simulink model "exercise02_simulation_model_template_R2025b_Solution"  (R2025b)
settings: Solver=FixedStepAuto  StartTime=0.0  StopTime=10.0  FixedStep=1e-5  RelTol=1e-3
PreLoadFcn:
  | exercise02_simulation_parameters
undefined symbols (not defined in the file or in its folder): g, nrotor_initial_conditions, nrotor_vehicle, reference, sigbuilder_block
settings Model: Creator=resjoehr  LastModifiedBy=diego
settings DataIOCC: SaveFormat=Array  StreamToWks=off  ReturnWorkspaceOutputs=off

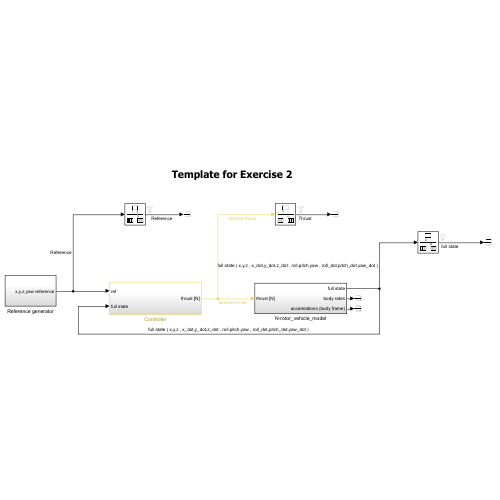
[thumbnail: Simulink's stored preview of the top-level diagram]
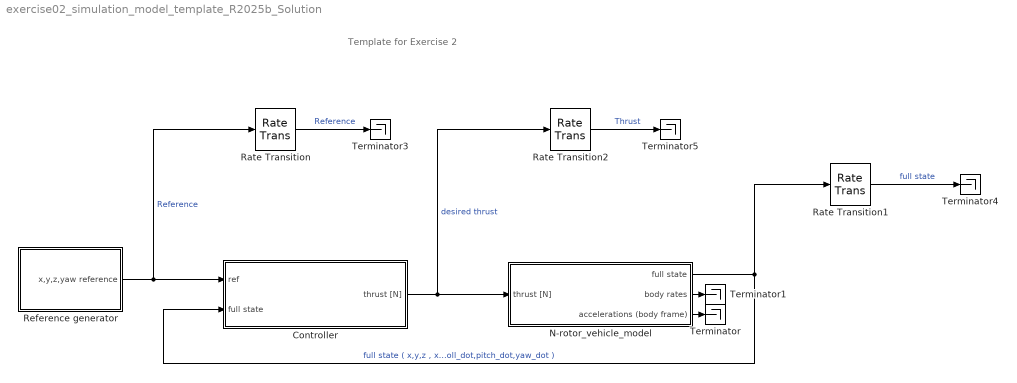
== system exercise02_simulation_model_template_R2025b_Solution ==
  note: Template for Exercise 2
  Controller : Subsystem
  N-rotor_vehicle_model : Subsystem
  Rate Transition : RateTransition  OutPortSampleTime=0.001
  Rate Transition1 : RateTransition  OutPortSampleTime=0.001
  Rate Transition2 : RateTransition  OutPortSampleTime=0.001
  Reference generator : Subsystem
  Terminator{,1,3..5} (5 alike) : Terminator
  wires:
  Rate Transition/1 -> Terminator3/1  "Reference"
  N-rotor_vehicle_model/2(body rates) -> Terminator1/1
  Reference generator/1(x,y,z,yaw reference) -> Rate Transition/1, Controller/1(ref)  "Reference"
  N-rotor_vehicle_model/1(full state) -> Rate Transition1/1, Controller/2(full state)  "full state ( x,y,z , x_dot,y_dot,z_dot , roll,pitch,yaw , roll_dot,pitch_dot,yaw_dot )"
  Rate Transition1/1 -> Terminator4/1  "full state"
  Rate Transition2/1 -> Terminator5/1  "Thrust"
  Controller/1(thrust [N]) -> N-rotor_vehicle_model/1(thrust [N]), Rate Transition2/1  "desired thrust"
  N-rotor_vehicle_model/3(accelerations (body frame)) -> Terminator/1

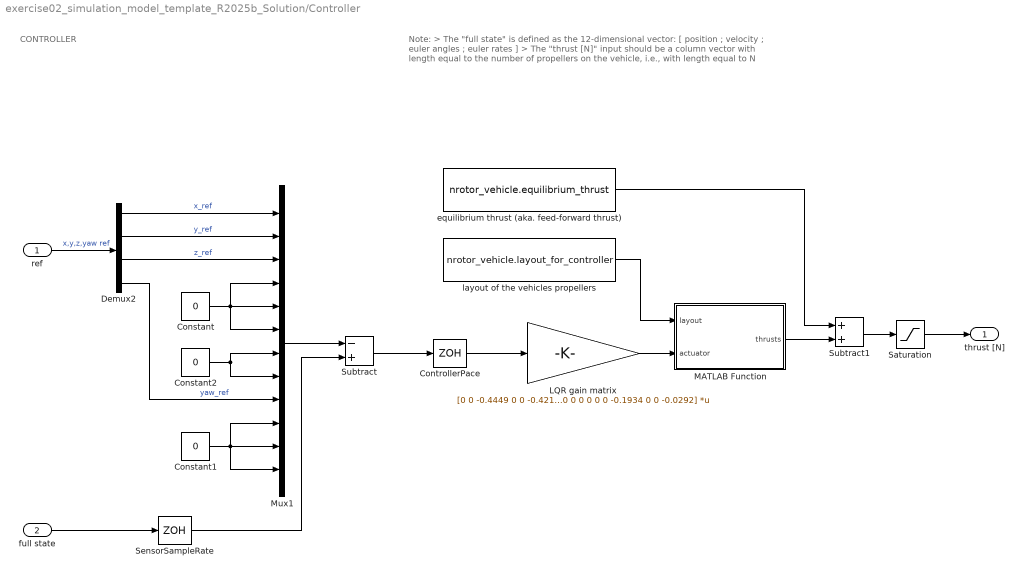
== system exercise02_simulation_model_template_R2025b_Solution/Controller ==
  note: CONTROLLER
  note: Note:
      | > The "full state" is defined as the 12-dimensional vector:
      | [ position ; velocity ; euler angles ; euler rates ]
      | > The "thrust [N]" input should be a column vector with
      | length equal to the number of propellers on the vehicle,
      | i.e., with length equal to N
  ref : Inport
  full state : Inport  Port=2
  Constant : Constant  Value=0
  Constant1 : Constant  Value=0
  Constant2 : Constant  Value=0
  ControllerPace : ZeroOrderHold  SampleTime=0.1
  Demux2 : Demux
  LQR gain matrix : Gain  Gain=[0 0 -0.4449 0 0 -0.4218 0 0 0 0 0 0;0 0.1322 0 0 0.1006 0 -0.3757 0 0 -0.0287 0 0;-0.1322 0 0 -0.1006 0 0 0 -0.3757 0 0 -0.0287 0;0 0 0 0 0 0 0 0 -0.1934 0 0 -0.0292]  Multiplication=Matrix(K*u)
  MATLAB Function : MATLAB Function  TreatAsAtomicUnit=on
  Mux1 : Mux  Inputs=12
  Saturation : Saturate  UpperLimit=nrotor_vehicle.thrust_max  LowerLimit=nrotor_vehicle.thrust_min  ZeroCross=off
  SensorSampleRate : ZeroOrderHold  SampleTime=0.005
  Subtract : Sum  Inputs=-+
  Subtract1 : Sum
  equilibrium thrust (aka. feed-forward thrust) : Constant  Value=nrotor_vehicle.equilibrium_thrust
  layout of the vehicles propellers : Constant  Value=nrotor_vehicle.layout_for_controller
  thrust [N] : Outport  VectorParamsAs1DForOutWhenUnconnected=off
  wires:
  Saturation/1 -> thrust [N]/1
  ref/1 -> Demux2/1  "x,y,z,yaw ref"
  Mux1/1 -> Subtract/1
  Demux2/1 -> Mux1/1  "x_ref"
  Demux2/2 -> Mux1/2  "y_ref"
  Demux2/3 -> Mux1/3  "z_ref"
  Constant/1 -> Mux1/6, Mux1/5, Mux1/4
  full state/1 -> SensorSampleRate/1
  Subtract/1 -> ControllerPace/1
  LQR gain matrix/1 -> MATLAB Function/2(actuator)
  Subtract1/1 -> Saturation/1
  equilibrium thrust (aka. feed-forward thrust)/1 -> Subtract1/1
  Constant1/1 -> Mux1/11, Mux1/12, Mux1/10
  Constant2/1 -> Mux1/8, Mux1/7
  Demux2/4 -> Mux1/9  "yaw_ref"
  MATLAB Function/1(thrusts) -> Subtract1/2
  layout of the vehicles propellers/1 -> MATLAB Function/1(layout)
  ControllerPace/1 -> LQR gain matrix/1
  SensorSampleRate/1 -> Subtract/2

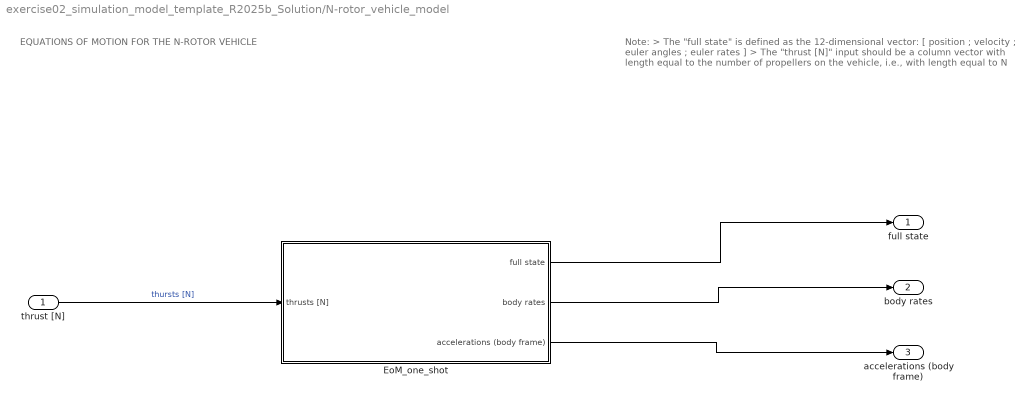
== system exercise02_simulation_model_template_R2025b_Solution/N-rotor_vehicle_model ==
  note: Note:
      | > The "full state" is defined as the 12-dimensional vector:
      | [ position ; velocity ; euler angles ; euler rates ]
      | > The "thrust [N]" input should be a column vector with
      | length equal to the number of propellers on the vehicle,
      | i.e., with length equal to N
  note: EQUATIONS OF MOTION FOR THE N-ROTOR VEHICLE
  thrust [N] : Inport
  EoM_one_shot : Subsystem
  full state : Outport  VectorParamsAs1DForOutWhenUnconnected=off
  body rates : Outport  Port=2  VectorParamsAs1DForOutWhenUnconnected=off
  accelerations (body frame) : Outport  Port=3  VectorParamsAs1DForOutWhenUnconnected=off
  wires:
  thrust [N]/1 -> EoM_one_shot/1(thrusts [N])  "thursts [N]"
  EoM_one_shot/1(full state) -> full state/1
  EoM_one_shot/2(body rates) -> body rates/1
  EoM_one_shot/3(accelerations (body frame)) -> accelerations (body frame)/1

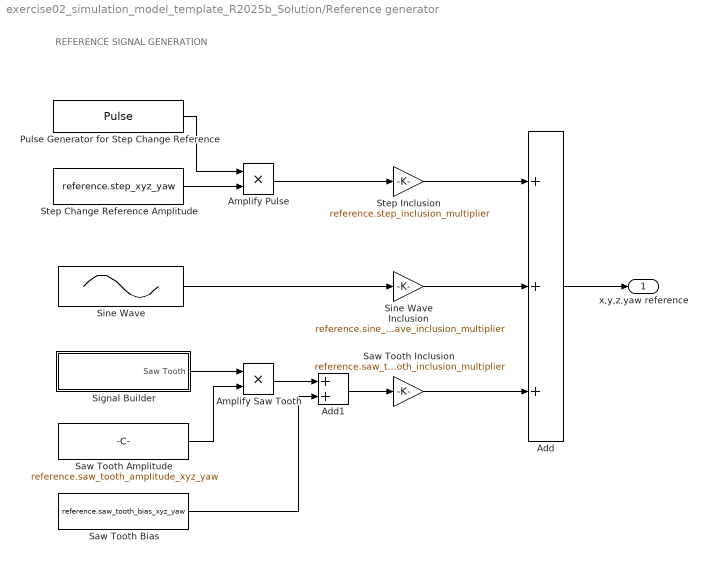
== system exercise02_simulation_model_template_R2025b_Solution/Reference generator ==
  note: REFERENCE SIGNAL GENERATION
  Add : Sum  Inputs=+++
  Add1 : Sum
  Amplify Pulse : Product
  Amplify Saw Tooth : Product
  Pulse Generator for Step Change Reference : DiscretePulseGenerator  PulseType=Time based  Period=reference.step_period*2  PulseWidth=50
  Saw Tooth Amplitude : Constant  Value=reference.saw_tooth_amplitude_xyz_yaw
  Saw Tooth Bias : Constant  Value=reference.saw_tooth_bias_xyz_yaw
  Saw Tooth Inclusion : Gain  Gain=reference.saw_tooth_inclusion_multiplier
  Signal Builder : Subsystem  Tag=STV Subsys  LoadFcn=sigbuilder_block('load');  StartFcn=sigbuilder_block('start');  StopFcn=sigbuilder_block('stop');  ClipboardFcn=sigbuilder_block('clipboard');  mask(Sigbuilder block){tuvar=[0:10]}
      mask help: Simulink:masks:SigbuilderBlock_MD
      mask init:
      | if ~strcmp(get_param(bdroot(gcbh),'SimulationStatus'),'stopped') tuvar = sigbuilder_block('maskInit'); end
      settings: CopyFcn=sigbuilder_block('copy');  DeleteFcn=sigbuilder_block('delete');  ModelCloseFcn=sigbuilder_block('modelClose');  PreSaveFcn=sigbuilder_block('preSave');  PauseFcn=sigbuilder_block('pause');  ContinueFcn=sigbuilder_block('continue');  NameChangeFcn=sigbuilder_block('namechange');  OpenFcn=sigbuilder_block('open',[1782.75 377.25 895.5 539.25 ]);  CloseFcn=sigbuilder_block('close');
      mask Display: plot(0, 0, 100, 100,[2, 2, 32, 32, 2], [68, 8, 8, 68, 68],[32, 2], [38, 38], [32, 19, 2],[53, 60, 44], [32, 17, 17, 2],[16, 16, 31, 31]);txt = getActiveGroup(gcbh);text(2, 100, txt,'verticalAlignment', 'top');
  Sine Wave : Sin  Amplitude=reference.sine_amplitude_xyz_yaw  Bias=reference.sine_bias_xyz_yaw  Frequency=2*pi()/reference.sine_period  SampleTime=0
  Sine Wave Inclusion : Gain  Gain=reference.sine_wave_inclusion_multiplier
  Step Change Reference Amplitude : Constant  Value=reference.step_xyz_yaw
  Step Inclusion : Gain  Gain=reference.step_inclusion_multiplier
  x,y,z,yaw reference : Outport  VectorParamsAs1DForOutWhenUnconnected=off
  wires:
  Step Change Reference Amplitude/1 -> Amplify Pulse/2
  Pulse Generator for Step Change Reference/1 -> Amplify Pulse/1
  Sine Wave/1 -> Sine Wave Inclusion/1
  Add/1 -> x,y,z,yaw reference/1
  Step Inclusion/1 -> Add/1
  Sine Wave Inclusion/1 -> Add/2
  Amplify Pulse/1 -> Step Inclusion/1
  Saw Tooth Inclusion/1 -> Add/3
  Signal Builder/1(Saw Tooth) -> Amplify Saw Tooth/1
  Saw Tooth Amplitude/1 -> Amplify Saw Tooth/2
  Amplify Saw Tooth/1 -> Add1/1
  Add1/1 -> Saw Tooth Inclusion/1
  Saw Tooth Bias/1 -> Add1/2

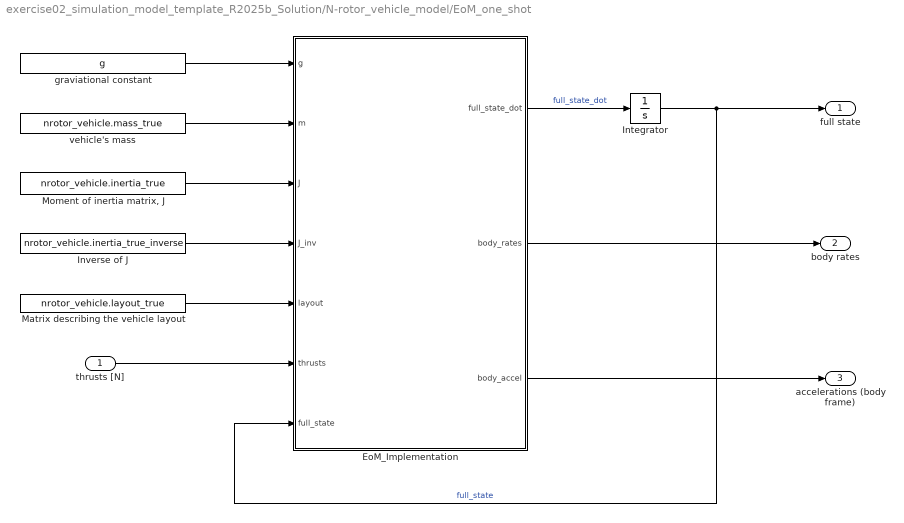
== system exercise02_simulation_model_template_R2025b_Solution/N-rotor_vehicle_model/EoM_one_shot ==
  thrusts [N] : Inport
  EoM_Implementation : MATLAB Function  TreatAsAtomicUnit=on
  Integrator : Integrator  InitialCondition=nrotor_initial_conditions
  Inverse of J : Constant  Value=nrotor_vehicle.inertia_true_inverse
  Matrix describing the vehicle layout : Constant  Value=nrotor_vehicle.layout_true
  "Moment of inertia matrix, J" : Constant  Value=nrotor_vehicle.inertia_true
  graviational constant : Constant  Value=g
  vehicle's mass : Constant  Value=nrotor_vehicle.mass_true
  full state : Outport  VectorParamsAs1DForOutWhenUnconnected=off
  body rates : Outport  Port=2  VectorParamsAs1DForOutWhenUnconnected=off
  accelerations (body frame) : Outport  Port=3  VectorParamsAs1DForOutWhenUnconnected=off
  wires:
  thrusts [N]/1 -> EoM_Implementation/6(thrusts)
  EoM_Implementation/2(body_rates) -> body rates/1
  Inverse of J/1 -> EoM_Implementation/4(J_inv)
  "Moment of inertia matrix, J"/1 -> EoM_Implementation/3(J)
  graviational constant/1 -> EoM_Implementation/1(g)
  vehicle's mass/1 -> EoM_Implementation/2(m)
  Matrix describing the vehicle layout/1 -> EoM_Implementation/5(layout)
  Integrator/1 -> EoM_Implementation/7(full_state), full state/1  "full_state"
  EoM_Implementation/1(full_state_dot) -> Integrator/1  "full_state_dot"
  EoM_Implementation/3(body_accel) -> accelerations (body frame)/1

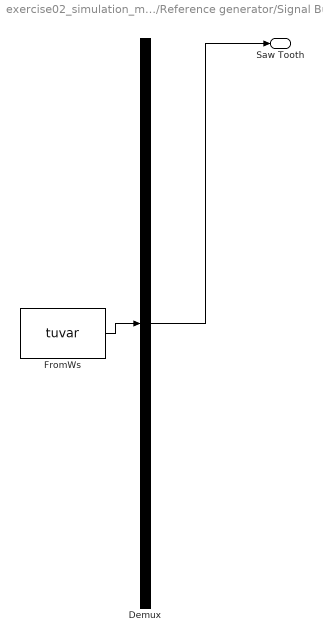
== system exercise02_simulation_model_template_R2025b_Solution/Reference generator/Signal Builder ==
  Demux : Demux  Tag=STV Demux  Outputs=1
      settings: DisplayOption=none
  FromWs : FromWorkspace  Tag=STV FromWs  VariableName=tuvar
      SigBuilderData=|
      | common.afterFinalStr = 'Extrapolate'
      | common.sampleTime = 0
      | dataSet.timeRange = [0 10]
      | dataSet.name = 'Group 1'
      | sbobj.Groups.Name = 'Group 1'
      | sbobj.Groups.Signals.Name = 'Saw Tooth'
      | sbobj.Groups.Signals.XData = [0 2.5 7.5 10]
      | sbobj.Groups.Signals.YData = [0 1.01 -1 0]
  Saw Tooth : Outport  Tag=STV Outport  VectorParamsAs1DForOutWhenUnconnected=off
  wires:
  Demux/1 -> Saw Tooth/1
  FromWs/1 -> Demux/1

== matlab function exercise02_simulation_model_template_R2025b_Solution/Controller/MATLAB Function ==
  data: layout input; actuator input; thrusts output
function thrusts = fcn(layout,actuator)

% INPUT ARGUMENTS:
% > actuator
%   This is the desired actuator values as requested by the "u=Kx"
%   computation where "K" is the LQR controller gain matrix
% > layout
%   This describes the layout of the N-rotor vehicle, following the usual
%   convention
%
% OUTPUT ARGUMENTS
% > thrusts
%   This is the adjustment thrusts to request from each propeller of the
%   N-rotor vehicle, i.e., this should be added to the equilibrium thrusts

% STEP 1:
% Construct the "propeller-force-to-actuator" conversion matrix:
nrotor_vehicle_M = [...
        ones(1,size(layout,2)) ;...
        layout(2,:) ;...
       -layout(1,:) ;...
        layout(3,:)  ...
    ];

% STEP 2:
% Second, compute the equilibrium thrust as the solution of the
% following minimisation problem:
%     
%     minimise       sum_{i=1}^{N} thrust_i^2
%
%     subject to:    nrotor_vehicle_M * [ thrust_1 ; ... ; thrust_N ] ...
%                          == [ total_force ; body_x_torque ; body_y_torque ; body_z_torque ]
%
%     For which the solution satisfies
%     [ eye(N) , nrotor_vehicle_M' ; nrotor_vehicle_M , zeros(4,4) ] ...
%                   == [ zeros(N,1) ; actuator ]
%

% Put the number of rotors into a variable with a shorter name:
nu = size(layout,2);

% Compute the solution:
temp_solution = ...
    [ eye(nu) , nrotor_vehicle_M' ; nrotor_vehicle_M , zeros(4,4) ] ...
        \ [ zeros(nu,1) ; actuator ];

% Extract the equilibrium thrusts from the solution
thrusts = temp_solution(1:nu,1);

== matlab function exercise02_simulation_model_template_R2025b_Solution/N-rotor_vehicle_model/EoM_one_shot/EoM_Implementation ==
  data: g input; full_state_dot output; m input; J input; J_inv input; layout input; thrusts input; full_state input; body_rates output; body_accel output
function [full_state_dot,body_rates,body_accel] = fcn_eom_template(g,m,J,J_inv,layout,thrusts,full_state)
%
% ----------------------------------------------------------------------- %
% DESCRIPTION:
% This function is a template for implementing the full equations of motion
% in one function.
%
%
% INPUT ARGUMENTS:
% m
% > This is the mass of the vehicle, in units of kilograms
%
% g
% > This is the acceleration due to gravity (typically 9.81), in units of
%   meters per second squared
%
% J
% > This is the moment of inertia matrix of the vehicle (it should be a
%   3-by3 matrix), the units of each element is kilogram meters squared
%
% J_inv
% > This is the inverse of the momement of inertia matrix, it is not
%   compute in this script to reduce the simulation run time slightly
%
% layout
% > This is a matrix that specifies the layout via the following format:
% nrotor_vehicle_layout = [...
%       x_1  ,  x_2  ,  ...  ,  x_{N-1}  ,  x_{N}  ;...
%       y_1  ,  y_2  ,  ...  ,  y_{N-1}  ,  y_{N}  ;...
%       c_1  ,  c_2  ,  ...  ,  c_{N-1}  ,  c_{N}   ...
%   ];
% where:
%   > x_i   is the x coordinate of propeller "i" relative to the CoG
%   > y_i   is the y coordinate of propeller "i" relative to the CoG
%   > c_i   is the thurst to torque coefficient of the propeller, with the
%           sign used to indicate the propeller's direction of rotation,
%           +ve indicates clock-wise propeller rotation.
%
% thrusts
% > This is a colulmn vector with length equal to the number of propellers
%   on the N-rotor vehicle, and each element represents the thrust force in
%   Newtons being produced by the respective propeller
%
% full_state
% > This is a vector of length 12 and is order as:
%   full_state[1:3]     the x,y,z posiiton of the body frame origin
%                       expressed in inertial frame coordinates, in units
%                       of [meters].
%
%   full_state[4:6]     the x,y,z linear velocity of the body frame origin
%                       expressed in inertial frame coordinates, in units
%                       of [meters per second].
%
%   full_state[7:9]     the roll, pitch, and yaw intrinsic Euler angles
%                       respectively, in units of [radians].
%
%   full_state[10:12]   the angular velocity of the roll, pitch, and yaw
%                       intrinsic Euler angles respectively, in units of
%                       [radians per second].
%
%
% RETURN ARGUMENTS:
% full_state_dot
% > This is a vector of length 12 and is ordered as:
%   full_state_dot[1:3]
%      - This is position dot and is taken directly as full_state[4:6]
%
%   full_state_dot[4:6]
%      - This is the position double dot and is computed using the equation
%        of motion for transaltion, it has units of [meters per second
%        squared]
%
%   full_state_dot[7:9]
%      - This is the angular velocity of the intrinsic Euler angles and is
%        taken directly as full_state[10:12]
%
%   full_state_dot[10:12]
%      - This is the angular accelerations of the intrinsic Euler angles
%        and is computed using the equation of motion for Euler angle
%        rotations, it has units of [radians per second squared]
%
% body_rates
% > This is a vector of length 3, each element represents the angular
%   velocity of the body frame as measured about the body frame's
%   coordinate axes, ordered as:
%   body_rates = [ w_x ; w_y ; w_z ];
%   In other words, this is exactly what is measured by a typical
%   strap-down Inertial Measurement Unit (IMU) that is attached to the body
%   of most all flying vehicles. It has units of [radians per second];
%
% body_accel
% > This is a vector of length 3, each element represents the linear
%   accelerations of the body frame as measured along the body frame's
%   coordinate axes, i.e., this is exctly what is measured by a typical
%   strap-down Inertial Measurement Unit (IMU). It is computed directly
%   from the "pos_double_dot" by applying the rotation matrix from inertial
%   to body frame. It has units of [meters per second squared].
%
% ----------------------------------------------------------------------- %


% Extract the components of the full state
pos      =  full_state(1:3);
pos_dot  =  full_state(4:6);
psi      =  full_state(7:9);
psi_dot  =  full_state(10:12);


% Extract each Euler angles
roll   =  psi(1);  % Roll  (gamma is the symbol used in the script)
pitch  =  psi(2);  % Pitch (beta  is the symbol used in the script)
yaw    =  psi(3);  % Yaw   (alpha is the symbol used in the script)


% Extract each Euler anglular rates
roll_dot   =  psi_dot(1);  % Roll  angular velocity
pitch_dot  =  psi_dot(2);  % Pitch angular velocity
yaw_dot    =  psi_dot(3); % Yaw   angular velocity, not needed





%% --------------------------------------------------------------------- %%
%% STUDENTS SHOULD EDIT THE FOLLOWING TO COMPLETE THE EQUATIONS OF MOTION
%  NOTE: Only the "R_B2I" and "T" matrices are already completed.


% Compute the rotation matrix from body frame to inertial frame:
R_B2I = [...
        cos(yaw)*cos(pitch)  ,...
            cos(yaw)*sin(pitch)*sin(roll)-sin(yaw)*cos(roll)  ,...
            cos(yaw)*sin(pitch)*cos(roll)+sin(yaw)*sin(roll)   ...
        ;...
        sin(yaw)*cos(pitch)  ,...
            sin(yaw)*sin(pitch)*sin(roll)+cos(yaw)*cos(roll)  ,...
            sin(yaw)*sin(pitch)*cos(roll)-cos(yaw)*sin(roll)   ...
        ;...
        -sin(pitch)  ,...
            cos(pitch)*sin(roll)  ,...
            cos(pitch)*cos(roll)   ...
    ];


% Compute the T matrix:
T = [...
        1  ,  0          ,  -sin(pitch)            ;...
        0  ,  cos(roll)  ,   sin(roll)*cos(pitch)  ;...
        0  , -sin(roll)  ,   cos(roll)*cos(pitch)   ...
    ];


% Compute the T inverse matrix:
T_inv = [...
        1  ,  sin(roll)*tan(pitch)  ,   cos(roll)*tan(pitch)  ;...
        0  ,  cos(roll)             ,   -sin(roll)  ;...
        0  ,  sin(roll)*sec(pitch)  ,   cos(roll)*sec(pitch)   ...
    ];


% Compute the time derivative of the T matrix:
T_dot = [...
        0  ,  0                    ,   -pitch_dot*cos(pitch)  ;...
        0  ,  -roll_dot*sin(roll)  ,   roll_dot*cos(roll)*cos(pitch) - pitch_dot*sin(roll)*sin(pitch)  ;...
        0  ,  -roll_dot*cos(roll)  ,   -roll_dot*sin(roll)*cos(pitch) - pitch_dot*cos(roll)*sin(pitch)   ...
    ];


% Implement the equation of motion for translation
pos_double_dot = (1/m)*(R_B2I*[0 ; 0 ; sum(thrusts)] + [0 ; 0 ; -m*g]);


% Compute the body rates from the Euler angluar rates
w = T*psi_dot;


% Implement the equation of motion for body frame 
sm_x = layout(1, :)*thrusts;
sm_y = layout(2, :)*thrusts;
sm_c = layout(3, :)*thrusts;
w_dot = J_inv*([sm_y ; -sm_x ; sm_c] - cross(w,J*w));


% Implement the equation of motion for Euler angle rotations
psi_double_dot = T_inv*(w_dot-T_dot*psi_dot);


%% STUDENTS SHOULD EDIT THE ABOVE TO COMPLETE THE EQUATIONS OF MOTION
%% --------------------------------------------------------------------- %%





% Put together the "full_state_dot" return variable
full_state_dot = [...
        pos_dot ;...
        pos_double_dot ;...
        psi_dot ;...
        psi_double_dot ...
    ];


% Put together the "body_rates" return variable
body_rates = w;


% Finally compute the accelerations in the body frame
% > by "simply" rotating the inertial frame linear accelerations, i.e.,
%   "pos_double_dot", from the inertial frame into the body frame
% > do you need to account for the fact that the body frame accelerations
%   are measured in a rotating frame?
body_accel = transpose(R_B2I) * psi_double_dot;


end
